simulink model "PActual"  (R2024b)
settings: configuration reference "STM32H7_Config" (kept outside this file)
settings Model: DataDictionary=Master_Dictionary.sldd  EnableAccessToBaseWorkspace=off  Creator=torni  LastModifiedBy=William
settings ConfigSetRef: SourceName=STM32H7_Config

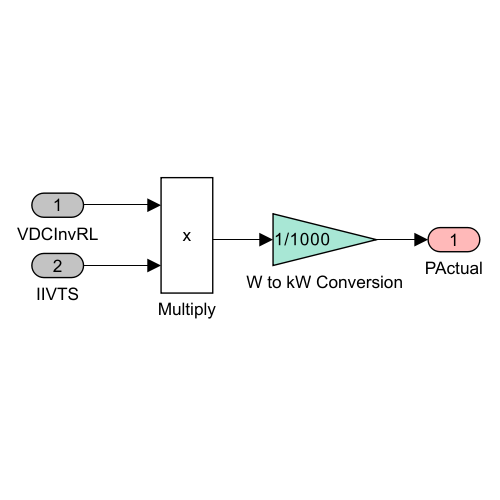
[thumbnail: Simulink's stored preview of the top-level diagram]
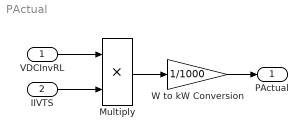
== system PActual ==
  VDCInvRL : Inport  OutDataTypeStr=double
  IIVTS : Inport  Port=2  OutDataTypeStr=double
  Multiply : Product
  W to kW Conversion : Gain  Gain=1/1000
  PActual : Outport  OutDataTypeStr=double  VectorParamsAs1DForOutWhenUnconnected=off
  wires:
  VDCInvRL/1 -> Multiply/1
  IIVTS/1 -> Multiply/2
  Multiply/1 -> W to kW Conversion/1
  W to kW Conversion/1 -> PActual/1
